simulink model "ThreePhHalfwaveSemiControlled"  (R2025a)
settings: Solver=VariableStepAuto  StartTime=0.0  StopTime=0.1  RelTol=1e-3
libraries: spsThyristorLib x3, spsCurrentMeasurementLib x1, spsDCVoltageSourceLib x1, spsDiodeLib x1, spsSeriesRLCBranchLib x1, spsThreePhaseVIMeasurementLib x1, spsThreePhaseSourceLib x1, spsVoltageMeasurementLib x1, sps_lib x1
settings Model: Creator=User  LastModifiedBy=samar

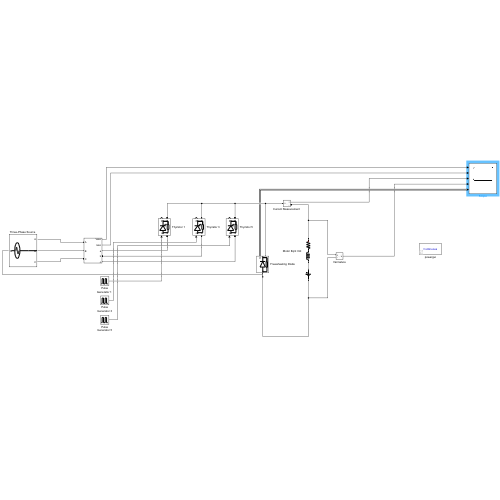
[thumbnail: Simulink's stored preview of the top-level diagram]
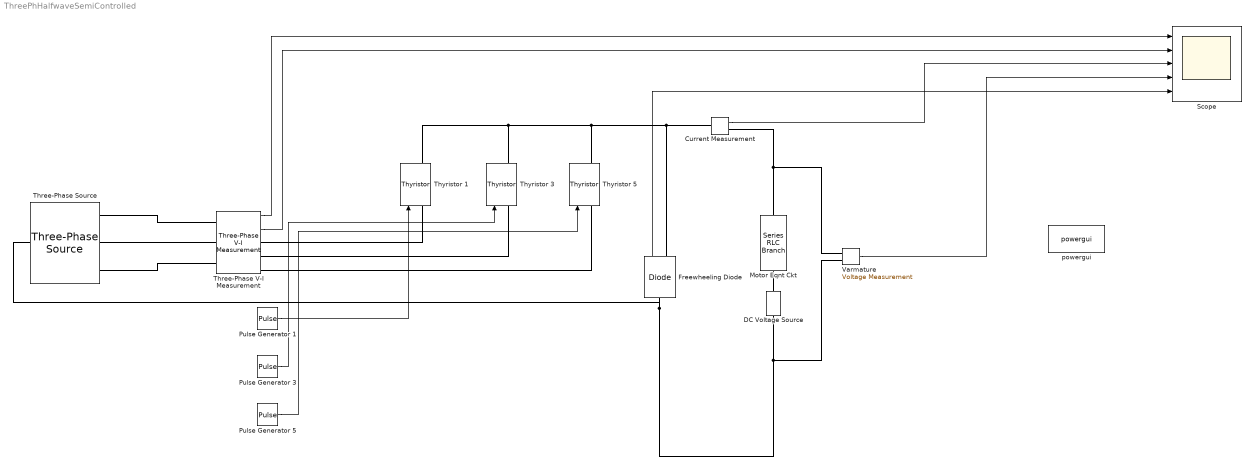
== system ThreePhHalfwaveSemiControlled ==
  "Current Measurement " : spsCurrentMeasurementLib/Current Measurement  PhasorSimulation=off  OutputType=Complex  PSBequivalent=0
  DC Voltage Source : spsDCVoltageSourceLib/DC Voltage Source  Amplitude=100  Measurements=Voltage
  Freewheeling Diode : spsDiodeLib/Diode  Ron=0.001  Lon=0  Vf=0.8  IC=0  UseSnubber=0  Rs=500  Cs=250e-9  Measurements=on
  Motor Eqnt Ckt : spsSeriesRLCBranchLib/Series RLC Branch  LConnTagsString=__new0  RConnTagsString=__new0  BranchType=RL  Resistance=1  Inductance=1e-3  SetiL0=off  InitialCurrent=0  Capacitance=1e-6  Setx0=off  InitialVoltage=0  Measurements=None
  "Pulse Generator 1 " : DiscretePulseGenerator  PulseType=Time based  Period=0.02  PulseWidth=5  PhaseDelay=0.00167
  Pulse Generator 3 : DiscretePulseGenerator  PulseType=Time based  Period=5  PulseWidth=5  PhaseDelay=0.00833
  Pulse Generator 5 : DiscretePulseGenerator  PulseType=Time based  Period=5  PulseWidth=5  PhaseDelay=0.015
  Scope : Scope  NumInputPorts=5
      settings: ActiveDisplayYMinimum=-439.00583117435178  ActiveDisplayYMaximum=414.81672938491636
  Three-Phase V-I Measurement : spsThreePhaseVIMeasurementLib/Three-Phase V-I Measurement  VoltageMeasurement=phase-to-phase  SetLabelV=off  LabelV=Vabc  Vpu=off  VpuLL=off  CurrentMeasurement=yes  SetLabelI=off  LabelI=Iabc  Ipu=off  Pbase=100e6  Vbase=500e3  OutputType=Complex  PhasorSimulation=off  PSBequivalent=0
  "Three-Phase Source " : spsThreePhaseSourceLib/Three-Phase Source  InternalConnection=Yn  VoltagePhases=off  Voltage=230  PhaseAngle=0  Voltage_phases=[25e3 25e3 25e3]/sqrt(3)  PhaseAngles_phases=[0 -120 +120]  Frequency=50  NonIdealSource=off  SpecifyImpedance=off  Resistance=0.8929  Inductance=16.58e-3  ShortCircuitLevel=100e6  BaseVoltage=25e3  XRratio=7  BusType=PV  Pref=10e3  Qref=0  Prefabc=[10e3, 10e3, 10e3]  Qrefabc=[0, 0, 0]  Qmin=-inf  Qmax=inf
  Thyristor 1 : spsThyristorLib/Thyristor  Ron=0.001  Lon=0  Vf=0.8  IC=0  Rs=500  Cs=250e-9  Measurements=on
  Thyristor 3 : spsThyristorLib/Thyristor  Ron=0.001  Lon=0  Vf=0.8  IC=0  Rs=500  Cs=250e-9  Measurements=on
  Thyristor 5 : spsThyristorLib/Thyristor  Ron=0.001  Lon=0  Vf=0.8  IC=0  Rs=500  Cs=250e-9  Measurements=on
  Varmature : spsVoltageMeasurementLib/Voltage Measurement  PhasorSimulation=off  OutputType=Complex  PSBequivalent=0
  powergui : sps_lib/powergui  Priority=1  SimulationMode=Continuous  SampleTime=50e-6  frequency=60  Iterations=50  frequencyindice=50  Pbase=100e6  ErrMax=1e-4  UnitsV=kV  UnitsW=MW  buscounter=0  FunctionMessages=off  echomessages=off  EnableUseOfTLC=off  CurrentSourceSwitches=off  DisableSnubberDevices=off  DisableRonSwitches=off  DisableVfSwitches=off  DisplayEquations=off  AutomaticDiscreteSolvers=off  SolverType=Tustin/Backward Euler (TBE)  Interpol=off  ExternalGateDelay=off  methode=off  Ts=100  x0status=blocks  SPID=on  SwTol=0  HookPort=off  NonlinearTolerance=1e-4  nMaxIteration=100  ContinueOnMaxIteration=off  RestoreLinks=warning  ResistiveCurrentMeasurement=off  Frange=[0:2:500]  Ylog=off  Xlog=on  ShowGrid=off  save=off  variable=ZData  structure=0  ZoomFFT=off  StartTime=0.0  cycles=1  DisplayStyle=1  fundamental=60  FreqAxis=off  MaxFrequency=1000  frequencyindicesteady=1  RmsSteady=1  display=off
  wires:
  "Pulse Generator 1 "/1 -> Thyristor 1/1
  Pulse Generator 3/1 -> Thyristor 3/1
  Pulse Generator 5/1 -> Thyristor 5/1
  Three-Phase V-I Measurement/1 -> Scope/1
  Varmature/1 -> Scope/4
  "Current Measurement "/1 -> Scope/3
  Three-Phase V-I Measurement/2 -> Scope/2
  Freewheeling Diode/1 -> Scope/5
  connections:
  "Three-Phase Source "/RConn1 -- Three-Phase V-I Measurement/LConn1
  Three-Phase V-I Measurement/RConn3 -- Thyristor 5/LConn1
  Thyristor 1/RConn1 -- Thyristor 3/RConn1 -- Thyristor 5/RConn1 -- Freewheeling Diode/RConn1 -- "Current Measurement "/LConn1
  Varmature/LConn1 -- "Current Measurement "/RConn1 -- Motor Eqnt Ckt/LConn1
  Three-Phase V-I Measurement/RConn2 -- Thyristor 3/LConn1
  Three-Phase V-I Measurement/RConn1 -- Thyristor 1/LConn1
  "Three-Phase Source "/RConn3 -- Three-Phase V-I Measurement/LConn3
  "Three-Phase Source "/RConn2 -- Three-Phase V-I Measurement/LConn2
  DC Voltage Source/RConn1 -- Motor Eqnt Ckt/RConn1
  Varmature/LConn2 -- Freewheeling Diode/LConn1 -- "Three-Phase Source "/LConn1 -- DC Voltage Source/LConn1
